simulink model "ArduCopter33StabilizeController"  (R2015b)
settings: Solver=VariableStepAuto  StartTime=0.0  StopTime=10.0  RelTol=1e-3
undefined symbols (not defined in the file): AC_ATTITUDE_RATE_RP_CONTROLLER_OUT_MAX, AC_ATTITUDE_RATE_YAW_CONTROLLER_OUT_MAX, AP_MOTORS_MAX_NUM_MOTORS, AP_MOTORS_THR_LOW_CMP_DEFAULT, AP_MOTORS_THST_MAX_DEFAULT, AP_MOTORS_YAW_HEADROOM_DEFAULT, ArduCopter, hover_throttle_pwm, init_eta, pitch_factor, RATE_PITCH_D, RATE_PITCH_FILT_HZ, RATE_PITCH_I, RATE_PITCH_IMAX, RATE_PITCH_P, RATE_ROLL_D, RATE_ROLL_FILT_HZ, RATE_ROLL_I, RATE_ROLL_IMAX, RATE_ROLL_P, RATE_YAW_D, RATE_YAW_FILT_HZ, RATE_YAW_I, RATE_YAW_IMAX, RATE_YAW_P, roll_factor, rpy_pwm_scalar, THR_MAX_DEFAULT, THR_MIN_DEFAULT, throttle_hover, throttle_pwm_scalar, THROTTLE_RADIO_LIM, yaw_factor
settings Model: Creator=jeremie  LastModifiedBy=jban039

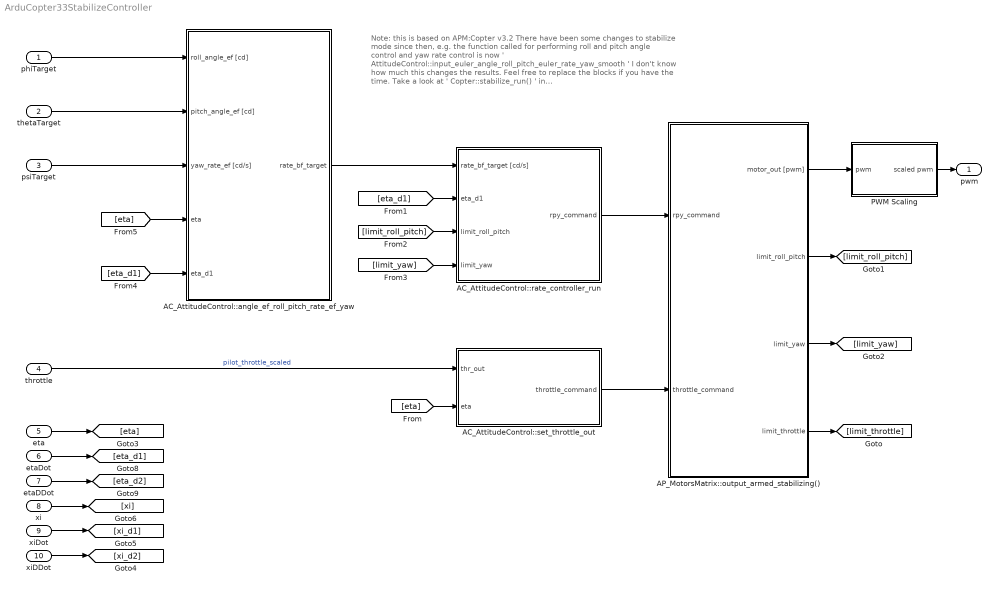
== system ArduCopter33StabilizeController ==
  note: Note: this is based on APM:Copter v3.2
      | There have been some changes to stabilize mode since then,
      | e.g. the function called for performing roll and pitch angle
      | control and yaw rate control is now
      | ' AttitudeControl::input_euler_angle_roll_pitch_euler_rate_yaw_smooth '
      | I don't know how much this changes the results. Feel free to replace the
      | blocks if you have the time.
      | Take a look at ' Copter::stabilize_run() ' in
      | ardupilot/Arducopter/control_stabilize.cpp and work from there.
  phiTarget : Inport
  thetaTarget : Inport  Port=2
  "psiTarget " : Inport  Port=3
  throttle : Inport  Port=4
  eta : Inport  Port=5
  etaDot : Inport  Port=6
  etaDDot : Inport  Port=7
  xi : Inport  Port=8
  xiDot : Inport  Port=9
  xiDDot : Inport  Port=10
  AC_AttitudeControl::angle_ef_roll_pitch_rate_ef_yaw : Subsystem
  AC_AttitudeControl::rate_controller_run : Subsystem
  AC_AttitudeControl::set_throttle_out : Subsystem
  AP_MotorsMatrix::output_armed_stabilizing() : Subsystem
  PWM Scaling : Subsystem
  pwm : Outport
  wires:
  AP_MotorsMatrix::output_armed_stabilizing()/1(motor_out [pwm]) -> PWM Scaling/1(pwm)
  xiDDot/1 -> [xi_d2]
  xiDot/1 -> [xi_d1]
  xi/1 -> [xi]
  AP_MotorsMatrix::output_armed_stabilizing()/2(limit_roll_pitch) -> [limit_roll_pitch]
  AP_MotorsMatrix::output_armed_stabilizing()/3(limit_yaw) -> [limit_yaw]
  AP_MotorsMatrix::output_armed_stabilizing()/4(limit_throttle) -> [limit_throttle]
  [eta] -> AC_AttitudeControl::set_throttle_out/2(eta)
  [eta_d1] -> AC_AttitudeControl::rate_controller_run/2(eta_d1)
  [limit_roll_pitch] -> AC_AttitudeControl::rate_controller_run/3(limit_roll_pitch)
  [limit_yaw] -> AC_AttitudeControl::rate_controller_run/4(limit_yaw)
  [eta] -> AC_AttitudeControl::angle_ef_roll_pitch_rate_ef_yaw/4(eta)
  AC_AttitudeControl::set_throttle_out/1(throttle_command) -> AP_MotorsMatrix::output_armed_stabilizing()/2(throttle_command)
  AC_AttitudeControl::rate_controller_run/1(rpy_command) -> AP_MotorsMatrix::output_armed_stabilizing()/1(rpy_command)
  etaDDot/1 -> [eta_d2]
  eta/1 -> [eta]
  etaDot/1 -> [eta_d1]
  AC_AttitudeControl::angle_ef_roll_pitch_rate_ef_yaw/1(rate_bf_target) -> AC_AttitudeControl::rate_controller_run/1(rate_bf_target [cd/s])
  [eta_d1] -> AC_AttitudeControl::angle_ef_roll_pitch_rate_ef_yaw/5(eta_d1)
  phiTarget/1 -> AC_AttitudeControl::angle_ef_roll_pitch_rate_ef_yaw/1(roll_angle_ef [cd])
  thetaTarget/1 -> AC_AttitudeControl::angle_ef_roll_pitch_rate_ef_yaw/2(pitch_angle_ef [cd])
  "psiTarget "/1 -> AC_AttitudeControl::angle_ef_roll_pitch_rate_ef_yaw/3(yaw_rate_ef [cd/s])
  throttle/1 -> AC_AttitudeControl::set_throttle_out/1(thr_out)  "pilot_throttle_scaled"
  PWM Scaling/1(scaled pwm) -> pwm/1

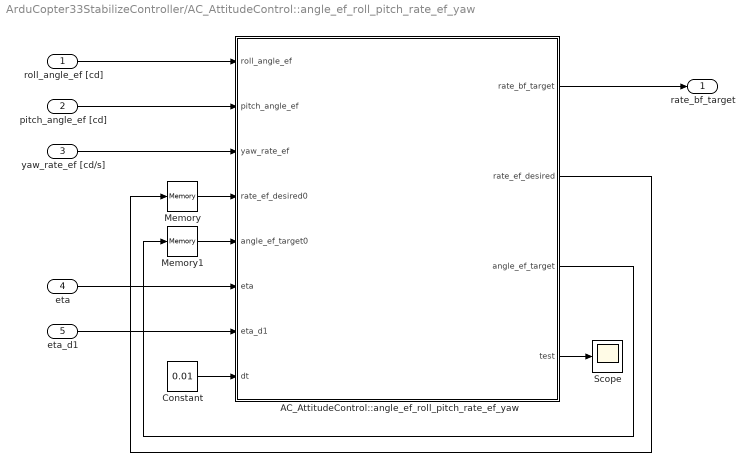
== system ArduCopter33StabilizeController/AC_AttitudeControl::angle_ef_roll_pitch_rate_ef_yaw ==
  roll_angle_ef [cd] : Inport
  pitch_angle_ef [cd] : Inport  Port=2
  yaw_rate_ef [cd/s] : Inport  Port=3
  eta : Inport  Port=4  PortDimensions=[3,1]
  eta_d1 : Inport  Port=5  PortDimensions=[3,1]
  AC_AttitudeControl::angle_ef_roll_pitch_rate_ef_yaw : MATLAB Function  TreatAsAtomicUnit=on  SystemSampleTime=0.01
  Constant : Constant  Value=0.01
  Memory : Memory  X0=[0;0;0]  InheritSampleTime=on
  Memory1 : Memory  X0=[0;0;init_eta(3)*180/pi*100]  InheritSampleTime=on
  Scope : Scope
  rate_bf_target : Outport
  wires:
  roll_angle_ef [cd]/1 -> AC_AttitudeControl::angle_ef_roll_pitch_rate_ef_yaw/1(roll_angle_ef)
  pitch_angle_ef [cd]/1 -> AC_AttitudeControl::angle_ef_roll_pitch_rate_ef_yaw/2(pitch_angle_ef)
  eta/1 -> AC_AttitudeControl::angle_ef_roll_pitch_rate_ef_yaw/6(eta)
  AC_AttitudeControl::angle_ef_roll_pitch_rate_ef_yaw/1(rate_bf_target) -> rate_bf_target/1
  AC_AttitudeControl::angle_ef_roll_pitch_rate_ef_yaw/4(test) -> Scope/1
  yaw_rate_ef [cd/s]/1 -> AC_AttitudeControl::angle_ef_roll_pitch_rate_ef_yaw/3(yaw_rate_ef)
  Memory/1 -> AC_AttitudeControl::angle_ef_roll_pitch_rate_ef_yaw/4(rate_ef_desired0)
  Memory1/1 -> AC_AttitudeControl::angle_ef_roll_pitch_rate_ef_yaw/5(angle_ef_target0)
  Constant/1 -> AC_AttitudeControl::angle_ef_roll_pitch_rate_ef_yaw/8(dt)
  AC_AttitudeControl::angle_ef_roll_pitch_rate_ef_yaw/2(rate_ef_desired) -> Memory/1
  AC_AttitudeControl::angle_ef_roll_pitch_rate_ef_yaw/3(angle_ef_target) -> Memory1/1
  eta_d1/1 -> AC_AttitudeControl::angle_ef_roll_pitch_rate_ef_yaw/7(eta_d1)

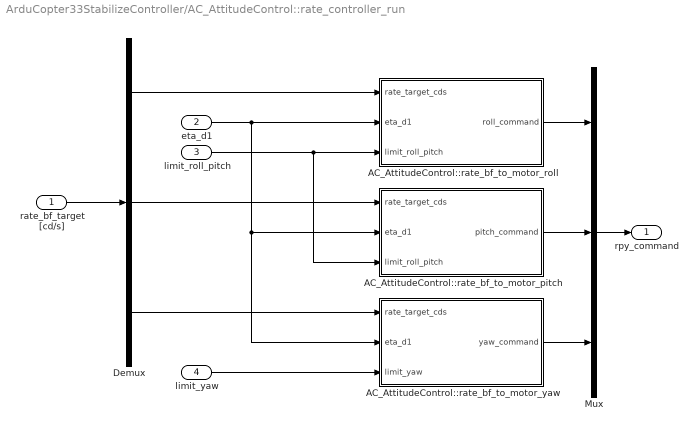
== system ArduCopter33StabilizeController/AC_AttitudeControl::rate_controller_run ==
  rate_bf_target [cd/s] : Inport
  eta_d1 : Inport  Port=2
  limit_roll_pitch : Inport  Port=3
  limit_yaw : Inport  Port=4
  AC_AttitudeControl::rate_bf_to_motor_pitch : Subsystem
  AC_AttitudeControl::rate_bf_to_motor_roll : Subsystem
  AC_AttitudeControl::rate_bf_to_motor_yaw : Subsystem
  Demux : Demux  Outputs=3
  Mux : Mux  Inputs=3
  rpy_command : Outport
  wires:
  eta_d1/1 -> AC_AttitudeControl::rate_bf_to_motor_yaw/2(eta_d1), AC_AttitudeControl::rate_bf_to_motor_pitch/2(eta_d1), AC_AttitudeControl::rate_bf_to_motor_roll/2(eta_d1)
  limit_yaw/1 -> AC_AttitudeControl::rate_bf_to_motor_yaw/3(limit_yaw)
  AC_AttitudeControl::rate_bf_to_motor_yaw/1(yaw_command) -> Mux/3
  AC_AttitudeControl::rate_bf_to_motor_pitch/1(pitch_command) -> Mux/2
  Mux/1 -> rpy_command/1
  AC_AttitudeControl::rate_bf_to_motor_roll/1(roll_command) -> Mux/1
  Demux/1 -> AC_AttitudeControl::rate_bf_to_motor_roll/1(rate_target_cds)
  Demux/2 -> AC_AttitudeControl::rate_bf_to_motor_pitch/1(rate_target_cds)
  Demux/3 -> AC_AttitudeControl::rate_bf_to_motor_yaw/1(rate_target_cds)
  rate_bf_target [cd/s]/1 -> Demux/1
  limit_roll_pitch/1 -> AC_AttitudeControl::rate_bf_to_motor_pitch/3(limit_roll_pitch), AC_AttitudeControl::rate_bf_to_motor_roll/3(limit_roll_pitch)

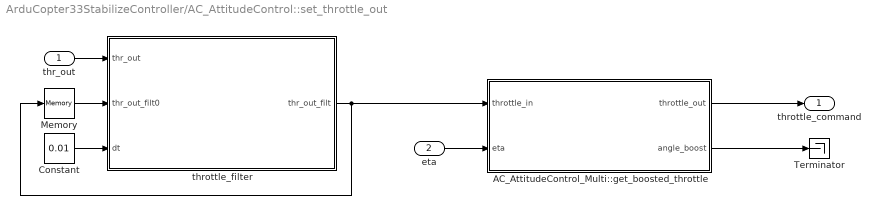
== system ArduCopter33StabilizeController/AC_AttitudeControl::set_throttle_out ==
  thr_out : Inport
  eta : Inport  Port=2
  AC_AttitudeControl_Multi::get_boosted_throttle : MATLAB Function  TreatAsAtomicUnit=on  SystemSampleTime=0.01
  Constant : Constant  Value=0.01
  Memory : Memory  X0=throttle_hover  InheritSampleTime=on
  Terminator : Terminator
  throttle_filter : MATLAB Function  TreatAsAtomicUnit=on  SystemSampleTime=0.01
  throttle_command : Outport
  wires:
  eta/1 -> AC_AttitudeControl_Multi::get_boosted_throttle/2(eta)
  AC_AttitudeControl_Multi::get_boosted_throttle/2(angle_boost) -> Terminator/1
  throttle_filter/1(thr_out_filt) -> Memory/1, AC_AttitudeControl_Multi::get_boosted_throttle/1(throttle_in)
  thr_out/1 -> throttle_filter/1(thr_out)
  Memory/1 -> throttle_filter/2(thr_out_filt0)
  Constant/1 -> throttle_filter/3(dt)
  AC_AttitudeControl_Multi::get_boosted_throttle/1(throttle_out) -> throttle_command/1

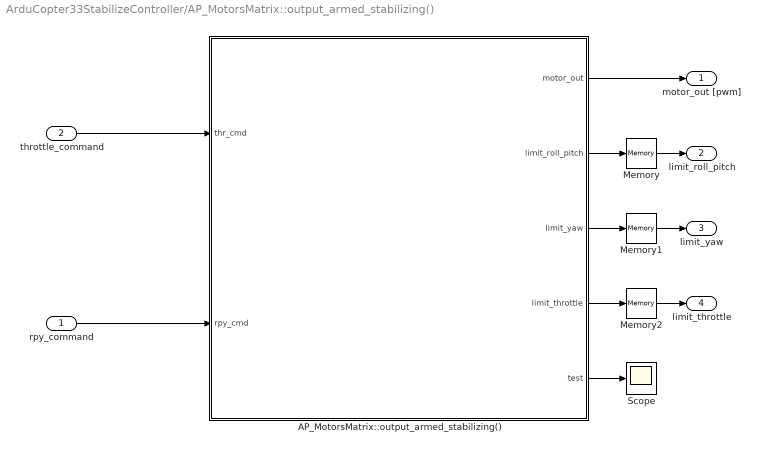
== system ArduCopter33StabilizeController/AP_MotorsMatrix::output_armed_stabilizing() ==
  rpy_command : Inport  PortDimensions=[3,1]
  throttle_command : Inport  Port=2
  AP_MotorsMatrix::output_armed_stabilizing() : MATLAB Function  TreatAsAtomicUnit=on  SystemSampleTime=0.01
  Memory : Memory  X0=false  InheritSampleTime=on
  Memory1 : Memory  X0=false  InheritSampleTime=on
  Memory2 : Memory  X0=boolean([0;0])  InheritSampleTime=on
  Scope : Scope
  motor_out [pwm] : Outport
  limit_roll_pitch : Outport  Port=2
  limit_yaw : Outport  Port=3
  limit_throttle : Outport  Port=4
  wires:
  AP_MotorsMatrix::output_armed_stabilizing()/1(motor_out) -> motor_out [pwm]/1
  rpy_command/1 -> AP_MotorsMatrix::output_armed_stabilizing()/2(rpy_cmd)
  AP_MotorsMatrix::output_armed_stabilizing()/5(test) -> Scope/1
  AP_MotorsMatrix::output_armed_stabilizing()/2(limit_roll_pitch) -> Memory/1
  AP_MotorsMatrix::output_armed_stabilizing()/3(limit_yaw) -> Memory1/1
  AP_MotorsMatrix::output_armed_stabilizing()/4(limit_throttle) -> Memory2/1
  throttle_command/1 -> AP_MotorsMatrix::output_armed_stabilizing()/1(thr_cmd)
  Memory/1 -> limit_roll_pitch/1
  Memory2/1 -> limit_throttle/1
  Memory1/1 -> limit_yaw/1

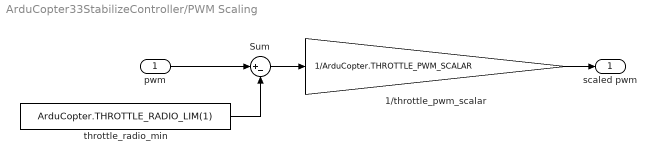
== system ArduCopter33StabilizeController/PWM Scaling ==
  pwm : Inport
  1/throttle_pwm_scalar : Gain  Gain=1/ArduCopter.THROTTLE_PWM_SCALAR
  Sum : Sum  Inputs=|+-
  throttle_radio_min : Constant  Value=ArduCopter.THROTTLE_RADIO_LIM(1)
  scaled pwm : Outport
  wires:
  1/throttle_pwm_scalar/1 -> scaled pwm/1
  throttle_radio_min/1 -> Sum/2
  Sum/1 -> 1/throttle_pwm_scalar/1
  pwm/1 -> Sum/1

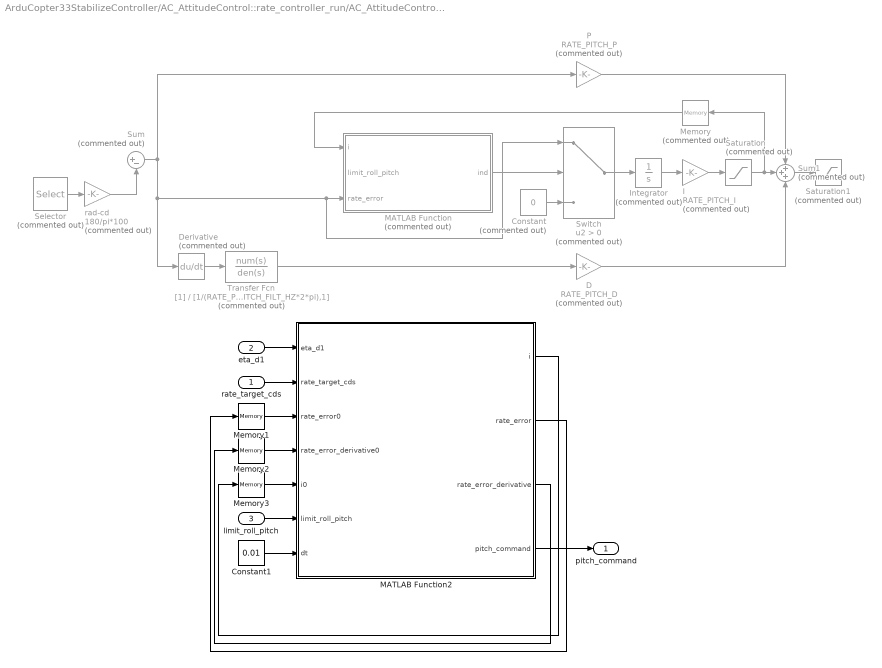
== system ArduCopter33StabilizeController/AC_AttitudeControl::rate_controller_run/AC_AttitudeControl::rate_bf_to_motor_pitch ==
  rate_target_cds : Inport
  eta_d1 : Inport  Port=2
  limit_roll_pitch : Inport  Port=3  OutDataTypeStr=boolean  PortDimensions=[1,1]
  Constant : Constant  Commented=on  Value=0
  Constant1 : Constant  Value=0.01
  D : Gain  Commented=on  Gain=RATE_PITCH_D
  Derivative : Derivative  Commented=on
  I : Gain  Commented=on  Gain=RATE_PITCH_I
  Integrator : Integrator  Commented=on
  MATLAB Function : MATLAB Function  Commented=on  TreatAsAtomicUnit=on
  MATLAB Function2 : MATLAB Function  TreatAsAtomicUnit=on  SystemSampleTime=0.01
  Memory : Memory  Commented=on  InheritSampleTime=on
  Memory1 : Memory  InheritSampleTime=on
  Memory2 : Memory  InheritSampleTime=on
  Memory3 : Memory  InheritSampleTime=on
  P : Gain  Commented=on  Gain=RATE_PITCH_P
  Saturation : Saturate  Commented=on  UpperLimit=RATE_PITCH_IMAX  LowerLimit=-RATE_PITCH_IMAX
  Saturation1 : Saturate  Commented=on  UpperLimit=AC_ATTITUDE_RATE_RP_CONTROLLER_OUT_MAX  LowerLimit=-AC_ATTITUDE_RATE_RP_CONTROLLER_OUT_MAX
  Selector : Selector  Commented=on  InputPortWidth=3  IndexOptions=Index vector (dialog)  Indices=2  OutputSizes=1
  Sum : Sum  Commented=on  Inputs=|+-
  Sum1 : Sum  Commented=on  Inputs=+++
  Switch : Switch  Commented=on  Criteria=u2 > Threshold
  Transfer Fcn : TransferFcn  Commented=on  Denominator=[1/(RATE_PITCH_FILT_HZ*2*pi),1]
  rad-cd : Gain  Commented=on  Gain=180/pi*100
  pitch_command : Outport
  wires:
  Memory1/1 -> MATLAB Function2/3(rate_error0)
  Memory3/1 -> MATLAB Function2/5(i0)
  MATLAB Function2/1(i) -> Memory3/1
  MATLAB Function2/2(rate_error) -> Memory1/1
  Constant1/1 -> MATLAB Function2/7(dt)
  Memory2/1 -> MATLAB Function2/4(rate_error_derivative0)
  MATLAB Function2/3(rate_error_derivative) -> Memory2/1
  rad-cd/1 -> Sum/2
  Integrator/1 -> I/1
  Derivative/1 -> Transfer Fcn/1
  I/1 -> Saturation/1
  Memory/1 -> MATLAB Function/1(i)
  Transfer Fcn/1 -> D/1
  Sum1/1 -> Saturation1/1
  P/1 -> Sum1/1
  D/1 -> Sum1/3
  Selector/1 -> rad-cd/1
  MATLAB Function/1(ind) -> Switch/2
  Sum/1 -> Derivative/1, Switch/1, MATLAB Function/3(rate_error), P/1
  Constant/1 -> Switch/3
  Saturation/1 -> Sum1/2, Memory/1
  Switch/1 -> Integrator/1
  MATLAB Function2/4(pitch_command) -> pitch_command/1
  limit_roll_pitch/1 -> MATLAB Function2/6(limit_roll_pitch)
  eta_d1/1 -> MATLAB Function2/1(eta_d1)
  rate_target_cds/1 -> MATLAB Function2/2(rate_target_cds)

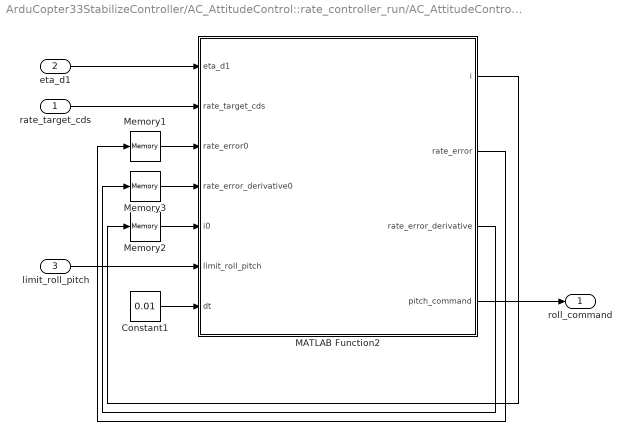
== system ArduCopter33StabilizeController/AC_AttitudeControl::rate_controller_run/AC_AttitudeControl::rate_bf_to_motor_roll ==
  rate_target_cds : Inport
  eta_d1 : Inport  Port=2
  limit_roll_pitch : Inport  Port=3  OutDataTypeStr=boolean  PortDimensions=[1,1]
  Constant1 : Constant  Value=0.01
  MATLAB Function2 : MATLAB Function  TreatAsAtomicUnit=on  SystemSampleTime=0.01
  Memory1 : Memory  InheritSampleTime=on
  Memory2 : Memory  InheritSampleTime=on
  Memory3 : Memory  InheritSampleTime=on
  roll_command : Outport
  wires:
  Memory1/1 -> MATLAB Function2/3(rate_error0)
  Memory2/1 -> MATLAB Function2/5(i0)
  MATLAB Function2/1(i) -> Memory2/1
  MATLAB Function2/2(rate_error) -> Memory1/1
  Constant1/1 -> MATLAB Function2/7(dt)
  Memory3/1 -> MATLAB Function2/4(rate_error_derivative0)
  MATLAB Function2/3(rate_error_derivative) -> Memory3/1
  MATLAB Function2/4(pitch_command) -> roll_command/1
  limit_roll_pitch/1 -> MATLAB Function2/6(limit_roll_pitch)
  eta_d1/1 -> MATLAB Function2/1(eta_d1)
  rate_target_cds/1 -> MATLAB Function2/2(rate_target_cds)

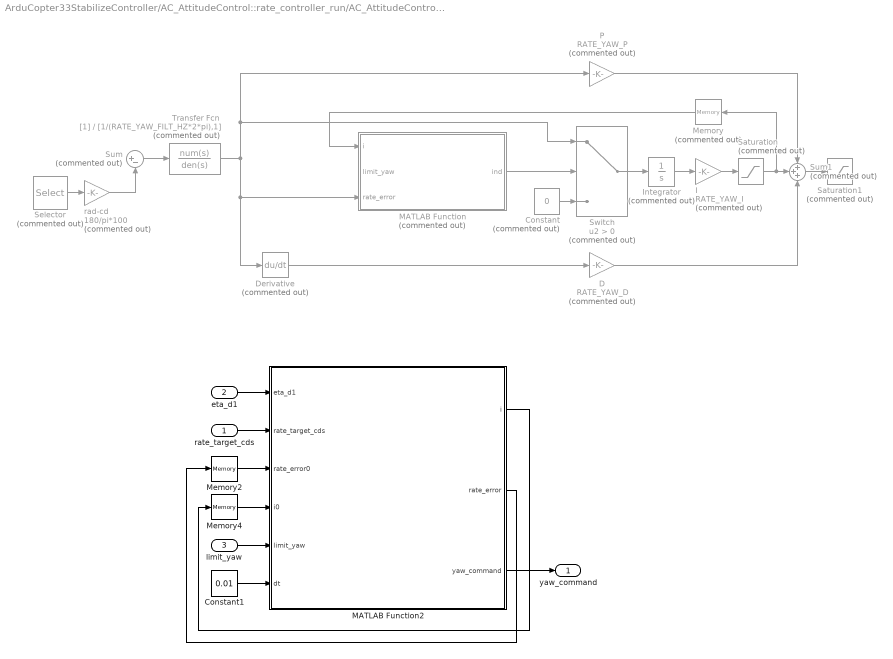
== system ArduCopter33StabilizeController/AC_AttitudeControl::rate_controller_run/AC_AttitudeControl::rate_bf_to_motor_yaw ==
  rate_target_cds : Inport
  eta_d1 : Inport  Port=2  PortDimensions=[3,1]
  limit_yaw : Inport  Port=3  OutDataTypeStr=boolean  PortDimensions=[1,1]
  Constant : Constant  Commented=on  Value=0
  Constant1 : Constant  Value=0.01
  D : Gain  Commented=on  Gain=RATE_YAW_D
  Derivative : Derivative  Commented=on
  I : Gain  Commented=on  Gain=RATE_YAW_I
  Integrator : Integrator  Commented=on
  MATLAB Function : MATLAB Function  Commented=on  TreatAsAtomicUnit=on
  MATLAB Function2 : MATLAB Function  TreatAsAtomicUnit=on  SystemSampleTime=0.01
  Memory : Memory  Commented=on  InheritSampleTime=on
  Memory2 : Memory  InheritSampleTime=on
  Memory4 : Memory  InheritSampleTime=on
  P : Gain  Commented=on  Gain=RATE_YAW_P
  Saturation : Saturate  Commented=on  UpperLimit=RATE_YAW_IMAX  LowerLimit=-RATE_YAW_IMAX
  Saturation1 : Saturate  Commented=on  UpperLimit=AC_ATTITUDE_RATE_YAW_CONTROLLER_OUT_MAX  LowerLimit=-AC_ATTITUDE_RATE_YAW_CONTROLLER_OUT_MAX
  Selector : Selector  Commented=on  InputPortWidth=3  IndexOptions=Index vector (dialog)  Indices=3  OutputSizes=1
  Sum : Sum  Commented=on  Inputs=|+-
  Sum1 : Sum  Commented=on  Inputs=+++
  Switch : Switch  Commented=on  Criteria=u2 > Threshold
  Transfer Fcn : TransferFcn  Commented=on  Denominator=[1/(RATE_YAW_FILT_HZ*2*pi),1]
  rad-cd : Gain  Commented=on  Gain=180/pi*100
  yaw_command : Outport
  wires:
  Memory2/1 -> MATLAB Function2/3(rate_error0)
  Memory4/1 -> MATLAB Function2/4(i0)
  Constant1/1 -> MATLAB Function2/6(dt)
  MATLAB Function2/1(i) -> Memory4/1
  MATLAB Function2/2(rate_error) -> Memory2/1
  rad-cd/1 -> Sum/2
  Integrator/1 -> I/1
  I/1 -> Saturation/1
  Memory/1 -> MATLAB Function/1(i)
  Derivative/1 -> D/1
  Sum1/1 -> Saturation1/1
  P/1 -> Sum1/1
  D/1 -> Sum1/3
  Selector/1 -> rad-cd/1
  MATLAB Function/1(ind) -> Switch/2
  Constant/1 -> Switch/3
  Saturation/1 -> Sum1/2, Memory/1
  Switch/1 -> Integrator/1
  Sum/1 -> Transfer Fcn/1
  Transfer Fcn/1 -> Derivative/1, MATLAB Function/3(rate_error), P/1, Switch/1
  limit_yaw/1 -> MATLAB Function2/5(limit_yaw)
  MATLAB Function2/3(yaw_command) -> yaw_command/1
  rate_target_cds/1 -> MATLAB Function2/2(rate_target_cds)
  eta_d1/1 -> MATLAB Function2/1(eta_d1)

== matlab function ArduCopter33StabilizeController/AC_AttitudeControl::set_throttle_out/AC_AttitudeControl_Multi::get_boosted_throttle ==
  data: throttle_in input; eta input; throttle_out output; THR_MIN_DEFAULT parameter; angle_boost output; throttle_pwm_scalar parameter
function [throttle_out,angle_boost] = get_boosted_throttle(throttle_in,eta,THR_MIN_DEFAULT,throttle_pwm_scalar)
%#codegen
min_throttle = THR_MIN_DEFAULT/throttle_pwm_scalar; % Is this correct?
cos_tilt = cos(eta(2))*cos(eta(1));
inverted_factor = constrain(2*cos_tilt,0,1);
boost_factor = 1/constrain(cos_tilt,0.5,1);

throttle_out = (throttle_in-min_throttle)*inverted_factor*boost_factor+min_throttle;
angle_boost = constrain(throttle_out-throttle_in,-32000,32000);

end

function constrain_val = constrain(val,min_val,max_val)
constrain_val = min([max([val,min_val]),max_val]);
end

== matlab function ArduCopter33StabilizeController/AC_AttitudeControl::angle_ef_roll_pitch_rate_ef_yaw/AC_AttitudeControl::angle_ef_roll_pitch_rate_ef_yaw ==
  data: roll_angle_ef input; pitch_angle_ef input; yaw_rate_ef input; rate_ef_desired0 input; angle_ef_target0 input; eta input; eta_d1 input; dt input; STABILIZE_ROLL_P parameter; STABILIZE_PITCH_P parameter; STABILIZE_YAW_P parameter; AC_ATTITUDE_CONTROL_ACCEL_RP_MAX_DEFAULT parameter; AC_ATTITUDE_ANGLE_CONTROLLER_ANGLE_MAX parameter; AC_ATTITUDE_CONTROL_ACCEL_Y_MAX_DEFAULT parameter; AC_ATTITUDE_ACCEL_RP_CONTROLLER_MIN parameter; AC_ATTITUDE_ACCEL_RP_CONTROLLER_MAX parameter; AC_ATTITUDE_ACCEL_Y_CONTROLLER_MIN parameter; AC_ATTITUDE_ACCEL_Y_CONTROLLER_MAX parameter; rate_bf_target output; rate_ef_desired output; angle_ef_target output; test output; AC_ATTITUDE_RATE_STAB_YAW_OVERSHOOT_ANGLE_MAX parameter
function [rate_bf_target,rate_ef_desired,angle_ef_target,test] = angle_ef_roll_pitch_rate_ef_yaw(roll_angle_ef,pitch_angle_ef,yaw_rate_ef,...
    rate_ef_desired0,angle_ef_target0,...
    eta,eta_d1,dt,...
    STABILIZE_ROLL_P,STABILIZE_PITCH_P,STABILIZE_YAW_P,...
    AC_ATTITUDE_CONTROL_ACCEL_RP_MAX_DEFAULT,...
    AC_ATTITUDE_ANGLE_CONTROLLER_ANGLE_MAX,AC_ATTITUDE_CONTROL_ACCEL_Y_MAX_DEFAULT,...
    AC_ATTITUDE_ACCEL_RP_CONTROLLER_MIN,AC_ATTITUDE_ACCEL_RP_CONTROLLER_MAX,...
    AC_ATTITUDE_ACCEL_Y_CONTROLLER_MIN,AC_ATTITUDE_ACCEL_Y_CONTROLLER_MAX,...
    AC_ATTITUDE_RATE_STAB_YAW_OVERSHOOT_ANGLE_MAX)
%#codegen
angle_kP = [STABILIZE_ROLL_P;
    STABILIZE_PITCH_P;
    STABILIZE_YAW_P];
accel_max = [AC_ATTITUDE_CONTROL_ACCEL_RP_MAX_DEFAULT;
    AC_ATTITUDE_CONTROL_ACCEL_RP_MAX_DEFAULT;
    AC_ATTITUDE_CONTROL_ACCEL_Y_MAX_DEFAULT];

% convert to centi-degrees
eta_cd = eta*(180/pi*100);

% initialise vectors
angle_ef_target = zeros(3,1); % [roll;pitch;yaw]
angle_ef_error = zeros(3,1);  % [roll;pitch;yaw]
rate_ef_desired = zeros(3,1);

% set earth-frame angle targets for roll and pitch and calculate angle error
angle_ef_target(1) = constrain(roll_angle_ef,-AC_ATTITUDE_ANGLE_CONTROLLER_ANGLE_MAX,AC_ATTITUDE_ANGLE_CONTROLLER_ANGLE_MAX);
angle_ef_error(1) = wrap_180_cd(angle_ef_target(1)-eta_cd(1));

angle_ef_target(2) = constrain(pitch_angle_ef,-AC_ATTITUDE_ANGLE_CONTROLLER_ANGLE_MAX,AC_ATTITUDE_ANGLE_CONTROLLER_ANGLE_MAX);
angle_ef_error(2) = wrap_180_cd(angle_ef_target(2)-eta_cd(2));

if (AC_ATTITUDE_CONTROL_ACCEL_Y_MAX_DEFAULT > 0)
    % set earth-frame feed forward rate for yaw
    rate_change_limit = AC_ATTITUDE_CONTROL_ACCEL_Y_MAX_DEFAULT*dt;
    rate_change = yaw_rate_ef-rate_ef_desired0(3);
    rate_change = constrain(rate_change,-rate_change_limit,rate_change_limit);
    rate_ef_desired(3) = rate_ef_desired0(3)+rate_change;
    % calculate yaw target angle and angle error
    [angle_ef_error(3),angle_ef_target(3)] = ...
        update_ef_yaw_angle_and_error(angle_ef_target0(3),...
        yaw_rate_ef,eta_cd(3),AC_ATTITUDE_RATE_STAB_YAW_OVERSHOOT_ANGLE_MAX,dt);
else
    % set yaw feed forward to zero
    rate_ef_desired(3) = yaw_rate_ef;
    % calculate yaw target angle and angle error
    [angle_ef_error(3),angle_ef_target(3)] = ...
        update_ef_yaw_angle_and_error(angle_ef_target0(3),...
        yaw_rate_ef,eta_cd(3),AC_ATTITUDE_RATE_STAB_YAW_OVERSHOOT_ANGLE_MAX,dt);
end
test = angle_ef_target0(3)-eta_cd(3);

% convert earth-frame angle errors to body-frame angle errors
angle_bf_error = frame_conversion_ef_to_bf(angle_ef_error,eta);

% convert body-frame angle errors to body-frame rate targets
rate_bf_target = update_rate_bf_targets(angle_bf_error,eta_d1,...
    angle_kP,accel_max,...
    AC_ATTITUDE_ACCEL_RP_CONTROLLER_MIN,AC_ATTITUDE_ACCEL_RP_CONTROLLER_MAX,...
    AC_ATTITUDE_ACCEL_Y_CONTROLLER_MIN,AC_ATTITUDE_ACCEL_Y_CONTROLLER_MAX); % CHECK YAW!!!

% set roll and pitch feed forward to zero
rate_ef_desired(1) = 0;
rate_ef_desired(2) = 0;

% convert earth-frame feed forward rates to body-frame feed forward rates
rate_bf_desired = frame_conversion_ef_to_bf(rate_ef_desired,eta);
rate_bf_target = rate_bf_target+rate_bf_desired;

end

%%
function constrain_val = constrain(val,min_val,max_val)
constrain_val = min([max([val,min_val]),max_val]);
end

function wrap_val = wrap_180_cd(val)
if (val > 360000 || val < -36000)
    % for very large numbers use modulus
    wrap_val = mod(val,36000);
else
    wrap_val = val;
end
while (wrap_val > 18000)
    wrap_val = wrap_val-36000;
end
while (wrap_val < -18000)
    wrap_val = wrap_val+36000;
end
end

function wrap_val = wrap_360_cd(val)
if (val >= 720000 || val < -360000)
    % for very large numbers use modulus
    wrap_val = mod(val,36000);
else
    wrap_val = val;
end
while (wrap_val >= 36000)
    wrap_val = wrap_val-36000;
end
while (wrap_val < 0)
    wrap_val = wrap_val+36000;
end
end

function [angle_ef_error_z,angle_ef_target_z] = update_ef_yaw_angle_and_error(angle_ef_target_z,yaw_rate_ef,yaw_sensor,overshoot_max,dt)
% calculate angle error with maximum of +- max angle overshoot
angle_ef_error_z = wrap_180_cd(angle_ef_target_z-yaw_sensor);
angle_ef_error_z = constrain(angle_ef_error_z,-overshoot_max,overshoot_max);

% update yaw angle target to be within max angle overshoot of our current heading
angle_ef_target_z = angle_ef_error_z+yaw_sensor;

% increment the yaw angle target
angle_ef_target_z = angle_ef_target_z+yaw_rate_ef*dt;
angle_ef_target_z = wrap_360_cd(angle_ef_target_z);
end

function bf_vector = frame_conversion_ef_to_bf(ef_vector,eta)
bf_vector = [1,0,-sin(eta(2));
    0,cos(eta(1)),sin(eta(1))*cos(eta(2));
    0,-sin(eta(1)),cos(eta(1))*cos(eta(2))]*ef_vector;
end

function rate_bf_target = update_rate_bf_targets(angle_bf_error,eta_d1,...
    angle_kP,accel_max,...
    AC_ATTITUDE_ACCEL_RP_CONTROLLER_MIN,AC_ATTITUDE_ACCEL_RP_CONTROLLER_MAX,...
    AC_ATTITUDE_ACCEL_Y_CONTROLLER_MIN,AC_ATTITUDE_ACCEL_Y_CONTROLLER_MAX)
rate_bf_target = zeros(3,1);

% stab roll calculation
% constrain roll rate request
rate_bf_target(1) = sqrt_controller(angle_bf_error(1),angle_kP(1),...
    constrain(accel_max(1)/2,AC_ATTITUDE_ACCEL_RP_CONTROLLER_MIN,AC_ATTITUDE_ACCEL_RP_CONTROLLER_MAX));

% stab pitch calculation
% constrain pitch rate request
rate_bf_target(2) = sqrt_controller(angle_bf_error(2),angle_kP(2),...
    constrain(accel_max(2)/2,AC_ATTITUDE_ACCEL_RP_CONTROLLER_MIN,AC_ATTITUDE_ACCEL_RP_CONTROLLER_MAX));

% stab yaw calculation
% constrain yaw rate request
rate_bf_target(3) = sqrt_controller(angle_bf_error(3),angle_kP(3),...
    constrain(accel_max(3)/2,AC_ATTITUDE_ACCEL_Y_CONTROLLER_MIN,AC_ATTITUDE_ACCEL_Y_CONTROLLER_MAX));

% include roll and pitch rate required to account for precession of the desired attitude about the body frame yaw axes
rate_bf_target(1) = rate_bf_target(1)+angle_bf_error(2)*eta_d1(3);
rate_bf_target(2) = rate_bf_target(2)-angle_bf_error(1)*eta_d1(3);
end

% AC_AttitudeControl::sqrt_controller
function u = sqrt_controller(error,p,second_ord_lim)
if (second_ord_lim == 0 || p == 0)
    u = error*p;
    return
end

linear_dist = second_ord_lim/p^2;

if (error > linear_dist)
    u = safe_sqrt(2*second_ord_lim*(error-(linear_dist/2)));
    return
elseif (error < -linear_dist)
    u = -safe_sqrt(2*second_ord_lim*(-error-(linear_dist/2)));
    return
else
    u = error*p;
    return
end
end

function v = safe_sqrt(u)
if (u < 0)
    v = 0;
else
    v = sqrt(u);
end
end

== matlab function ArduCopter33StabilizeController/AC_AttitudeControl::rate_controller_run/AC_AttitudeControl::rate_bf_to_motor_pitch/MATLAB Function2 ==
  data: eta_d1 input; i output; rate_target_cds input; rate_error0 input; rate_error_derivative0 input; i0 input; limit_roll_pitch input; rate_error output; rate_error_derivative output; pitch_command output; dt input; RATE_PITCH_P parameter; RATE_PITCH_I parameter; RATE_PITCH_D parameter; AC_ATTITUDE_RATE_RP_CONTROLLER_OUT_MAX parameter; RATE_PITCH_IMAX parameter; RATE_PITCH_FILT_HZ parameter
function [i,rate_error,rate_error_derivative,pitch_command] = ...
    rate_bf_to_motor_pitch(eta_d1,rate_target_cds,...
    rate_error0,rate_error_derivative0,i0,limit_roll_pitch,dt,...
    RATE_PITCH_P,RATE_PITCH_I,RATE_PITCH_D,AC_ATTITUDE_RATE_RP_CONTROLLER_OUT_MAX,...
    RATE_PITCH_IMAX,RATE_PITCH_FILT_HZ)
%#codegen

% get current rate
current_rate = eta_d1(2)*(180/pi*100); % BODY OR EARTH FRAME?

% calculate error and call pid controller
rate_error = rate_target_cds-current_rate;

% calculate and filter derivative
rate_error_derivative = set_input_filter_d(rate_error,rate_error0,rate_error_derivative0,RATE_PITCH_FILT_HZ,dt);

% get p value
p = RATE_PITCH_P*rate_error;

% get i term
i = i0;

% update i term as long as we haven't breached the limits or the i term
% will certainly reduce
if (~limit_roll_pitch || ((i > 0 && rate_error < 0) || (i < 0 && rate_error > 0)))
    i = get_i(RATE_PITCH_I,i,rate_error,RATE_PITCH_IMAX,dt);
end

% get d value
d = RATE_PITCH_D*rate_error_derivative;

% constrain output and return
pitch_command = constrain(p+i+d,-AC_ATTITUDE_RATE_RP_CONTROLLER_OUT_MAX,AC_ATTITUDE_RATE_RP_CONTROLLER_OUT_MAX);

end

%%
function con_val = constrain(val,min_val,max_val)
con_val = min([max([val,min_val]),max_val]);
end

function i = get_i(ki,i0,error,imax,dt)
i = i0+ki*error*dt;
if (i < -imax)
    i = -imax;
elseif (i > imax)
    i = imax;
end
end

function derivative = set_input_filter_d(input,input0,derivative0,filt_cutoff,dt)
rc = 1/(2*pi*filt_cutoff);
alpha = dt/(dt+rc);
derivative = (input-input0)/dt;
derivative = derivative0+alpha*(derivative-derivative0);
end

== matlab function ArduCopter33StabilizeController/AC_AttitudeControl::rate_controller_run/AC_AttitudeControl::rate_bf_to_motor_yaw/MATLAB Function2 ==
  data: eta_d1 input; i output; rate_target_cds input; rate_error0 input; i0 input; limit_yaw input; dt input; RATE_YAW_P parameter; RATE_YAW_I parameter; RATE_YAW_D parameter; rate_error output; yaw_command output; AC_ATTITUDE_RATE_YAW_CONTROLLER_OUT_MAX parameter; RATE_YAW_IMAX parameter; RATE_YAW_FILT_HZ parameter
function [i,rate_error,yaw_command] = ...
    rate_bf_to_motor_yaw(eta_d1,rate_target_cds,rate_error0,i0,limit_yaw,dt,...
    RATE_YAW_P,RATE_YAW_I,RATE_YAW_D,AC_ATTITUDE_RATE_YAW_CONTROLLER_OUT_MAX,...
    RATE_YAW_IMAX,RATE_YAW_FILT_HZ)
%#codegen

% get current rate
current_rate = eta_d1(3)*(180/pi*100); % BODY OR EARTH FRAME?

% calculate error and call pid controller
rate_error = rate_target_cds-current_rate;

% filter rate_error and calculate derivative
[rate_error,derivative_error] = set_input_filter_all(rate_error,rate_error0,RATE_YAW_FILT_HZ,dt);

% get p value
p = RATE_YAW_P*rate_error;

% get i term
i = i0;

% update i term as long as we haven't breached the limits or the i term
% will certainly reduce
if (~limit_yaw || ((i > 0 && rate_error < 0) || (i < 0 && rate_error > 0)))
    i = get_i(RATE_YAW_I,i,rate_error,RATE_YAW_IMAX,dt);
end

% get d value
d = RATE_YAW_D*derivative_error;

% constrain output and return
yaw_command = constrain(p+i+d,-AC_ATTITUDE_RATE_YAW_CONTROLLER_OUT_MAX,AC_ATTITUDE_RATE_YAW_CONTROLLER_OUT_MAX);

end

%%
function con_val = constrain(val,min_val,max_val)
con_val = min([max([val,min_val]),max_val]);
end

function i = get_i(ki,i0,error,imax,dt)
i = i0+ki*error*dt;
if (i < -imax)
    i = -imax;
elseif (i > imax)
    i = imax;
end
end

function [output,derivative] = set_input_filter_all(input,input0,filt_cutoff,dt)
rc = 1/(2*pi*filt_cutoff);
alpha = dt/(dt+rc);
input_filt_change = alpha*(input-input0);
output = input0+input_filt_change;
derivative = input_filt_change/dt;
end

== matlab function ArduCopter33StabilizeController/AC_AttitudeControl::rate_controller_run/AC_AttitudeControl::rate_bf_to_motor_pitch/MATLAB Function ==
  data: i input; ind output; limit_roll_pitch input; rate_error input
function ind = check_limits(i,limit_roll_pitch,rate_error)
%#codegen
ind = 0;
if (~limit_roll_pitch || ((i > 0 && rate_error < 0) || (i < 0 && rate_error > 0)))
   ind = 1; 
end
end

== matlab function ArduCopter33StabilizeController/AC_AttitudeControl::rate_controller_run/AC_AttitudeControl::rate_bf_to_motor_yaw/MATLAB Function ==
  data: i input; ind output; limit_yaw input; rate_error input
function ind = check_limits(i,limit_yaw,rate_error)
%#codegen
ind = 0;
if (~limit_yaw || ((i > 0 && rate_error < 0) || (i < 0 && rate_error > 0)))
   ind = 1; 
end
end

== matlab function ArduCopter33StabilizeController/AC_AttitudeControl::set_throttle_out/throttle_filter ==
  data: thr_out input; thr_out_filt0 input; dt input; POSCONTROL_THROTTLE_CUTOFF_FREQ parameter; thr_out_filt output
function thr_out_filt = fcn(thr_out,thr_out_filt0,dt,POSCONTROL_THROTTLE_CUTOFF_FREQ)
%#codegen
% Calculate alpha
rc = 1/(2*pi*POSCONTROL_THROTTLE_CUTOFF_FREQ);
alpha = dt/(dt+rc);
thr_out_filt = thr_out_filt0+alpha*double(thr_out-thr_out_filt0);
end

== matlab function ArduCopter33StabilizeController/AC_AttitudeControl::rate_controller_run/AC_AttitudeControl::rate_bf_to_motor_roll/MATLAB Function2 ==
  data: eta_d1 input; i output; rate_target_cds input; rate_error0 input; rate_error_derivative0 input; i0 input; limit_roll_pitch input boolean size=[1,1]; rate_error output; rate_error_derivative output; pitch_command output; dt input; RATE_ROLL_P parameter; RATE_ROLL_I parameter; RATE_ROLL_D parameter; AC_ATTITUDE_RATE_RP_CONTROLLER_OUT_MAX parameter; RATE_ROLL_IMAX parameter; RATE_ROLL_FILT_HZ parameter
function [i,rate_error,rate_error_derivative,pitch_command] = ...
    rate_bf_to_motor_roll(eta_d1,rate_target_cds,...
    rate_error0,rate_error_derivative0,i0,limit_roll_pitch,dt,...
    RATE_ROLL_P,RATE_ROLL_I,RATE_ROLL_D,AC_ATTITUDE_RATE_RP_CONTROLLER_OUT_MAX,...
    RATE_ROLL_IMAX,RATE_ROLL_FILT_HZ)
%#codegen

% get current rate
current_rate = eta_d1(1)*(180/pi*100); % BODY OR EARTH FRAME?

% calculate error and call pid controller
rate_error = rate_target_cds-current_rate;

% calculate and filter derivative
rate_error_derivative = set_input_filter_d(rate_error,rate_error0,rate_error_derivative0,RATE_ROLL_FILT_HZ,dt);

% get p value
p = RATE_ROLL_P*rate_error;

% get i term
i = i0;

% update i term as long as we haven't breached the limits or the i term
% will certainly reduce
if (~limit_roll_pitch || ((i > 0 && rate_error < 0) || (i < 0 && rate_error > 0)))
    i = get_i(RATE_ROLL_I,i,rate_error,RATE_ROLL_IMAX,dt);
end

% get d value
d = RATE_ROLL_D*rate_error_derivative;

% constrain output and return
pitch_command = constrain(p+i+d,-AC_ATTITUDE_RATE_RP_CONTROLLER_OUT_MAX,AC_ATTITUDE_RATE_RP_CONTROLLER_OUT_MAX);

end

%%
function con_val = constrain(val,min_val,max_val)
con_val = min([max([val,min_val]),max_val]);
end

function i = get_i(ki,i0,error,imax,dt)
i = i0+ki*error*dt;
if (i < -imax)
    i = -imax;
elseif (i > imax)
    i = imax;
end
end

function derivative = set_input_filter_d(input,input0,derivative0,filt_cutoff,dt)
rc = 1/(2*pi*filt_cutoff);
alpha = dt/(dt+rc);
derivative = (input-input0)/dt;
derivative = derivative0+alpha*(derivative-derivative0);
end

== matlab function ArduCopter33StabilizeController/AP_MotorsMatrix::output_armed_stabilizing()/AP_MotorsMatrix::output_armed_stabilizing() ==
  data: thr_cmd input; rpy_cmd input; THROTTLE_RADIO_LIM parameter; THR_MIN_DEFAULT parameter; THR_MAX_DEFAULT parameter; AP_MOTORS_THR_LOW_CMP_DEFAULT parameter; AP_MOTORS_YAW_HEADROOM_DEFAULT parameter; hover_throttle_pwm parameter; motor_out output size=4; throttle_pwm_scalar parameter size=1; rpy_pwm_scalar parameter; roll_factor parameter; pitch_factor parameter; yaw_factor parameter; limit_roll_pitch output; limit_yaw output; limit_throttle output; AP_MOTORS_THST_MAX_DEFAULT parameter; AP_MOTORS_MAX_NUM_MOTORS parameter; test output
function [motor_out,limit_roll_pitch, limit_yaw,limit_throttle,test]...
    = output_armed_stabilizing(thr_cmd,rpy_cmd,...
    THROTTLE_RADIO_LIM,THR_MIN_DEFAULT,THR_MAX_DEFAULT,AP_MOTORS_THR_LOW_CMP_DEFAULT,...
    AP_MOTORS_YAW_HEADROOM_DEFAULT,...
    hover_throttle_pwm,...
    throttle_pwm_scalar,rpy_pwm_scalar,...
    roll_factor,pitch_factor,yaw_factor,...
    AP_MOTORS_THST_MAX_DEFAULT,...
    AP_MOTORS_MAX_NUM_MOTORS)
%#codegen
throttle_radio_min = THROTTLE_RADIO_LIM(1);
throttle_radio_max = THROTTLE_RADIO_LIM(2);
min_throttle = THR_MIN_DEFAULT;
max_throttle = THR_MAX_DEFAULT;
%fx_factor = fxy_factor(:,1);
%fy_factor = fxy_factor(:,2);
throttle_thr_mix = AP_MOTORS_THR_LOW_CMP_DEFAULT;
yaw_headroom = AP_MOTORS_YAW_HEADROOM_DEFAULT;
thrust_curve_max = AP_MOTORS_THST_MAX_DEFAULT;
lift_max = 1;

% -------------------------------------------------------------------------
out_min_pwm = throttle_radio_min+min_throttle;
% out_min_pwm = throttle_radio_min+min_throttle*throttle_pwm_scalar; % JC: Alternative calculation?
out_max_pwm = throttle_radio_max;
out_mid_pwm = (out_min_pwm+out_max_pwm)/2;
rpy_scale = 1;              % This is used to scale the roll, pitch and yaw to fit within the motor limits

thr_adj = 0;        % The difference between the pilot's desired throttle and out_best_thr_pwm (the throttle that is actually provided) % WHERE IS THIS CALCULATED - CHECK!!!

% Initialise limit flags
limit_roll_pitch = false;
limit_yaw = false;
limit_throttle = false(2,1); % [lower,upper]

% Ensure throttle is within bounds of 0 to 1000
thr_in_min = rel_pwm_to_thr_range(min_throttle,throttle_pwm_scalar);
% thr_in_min = min_throttle; % Limit thr_cmd to 130-1000?
if (thr_cmd <= thr_in_min)
    thr_cmd = thr_in_min;
    limit_throttle(1) = true;
end
if (thr_cmd >= max_throttle)
    thr_cmd = max_throttle;
    limit_throttle(2) = true;
end

roll_pwm = rpy_cmd(1)*rpy_pwm_scalar;
pitch_pwm = rpy_cmd(2)*rpy_pwm_scalar;
yaw_pwm = rpy_cmd(3)*rpy_pwm_scalar;
throttle_radio_output = thr_cmd*throttle_pwm_scalar+throttle_radio_min;
%fx_pwm = fxy_cmd(1)*fxy_pwm_scalar;
%fy_pwm = fxy_cmd(2)*fxy_pwm_scalar;

% Calculate roll and pitch for each motor
rpy_out = roll_pwm*roll_factor+pitch_pwm*pitch_factor;
% Add fxy command for each motor
% rpy_out = rpy_out+fx_pwm*fx_factor+fy_pwm*fy_factor;
% Record high/low command
rpy_low = min(rpy_out);
rpy_high = max(rpy_out);

% KS: bypass this adjustment of throttle - need to resolve why only out_mid_pwm is the output for high input throttle settings
% calculate throttle that gives most possible room for yaw (range 1000 ~ 2000) which is the lower of:
%      1. mid throttle - average of highest and lowest motor (this would give the maximum possible room margin above the highest motor and below the lowest)
%      2. the higher of:
%            a) the pilot's throttle input
%            b) the mid point between the pilot's input throttle and hover-throttle
%      Situation #2 ensure we never increase the throttle above hover throttle unless the pilot has commanded this.
%      Situation #2b allows us to raise the throttle above what the pilot commanded but not so far that it would actually cause the copter to rise.
%      We will choose #1 (the best throttle for yaw control) if that means reducing throttle to the motors (i.e. we favour reducing throttle *because* it provides better yaw control)
%      We will choose #2 (a mix of pilot and hover throttle) only when the throttle is quite low.  We favour reducing throttle instead of better yaw control because the pilot has commanded it
motor_mid = (rpy_low+rpy_high)/2;
out_best_thr_pwm = min([out_mid_pwm-motor_mid,...
    max([throttle_radio_output,...
    throttle_radio_output*max([0,1-throttle_thr_mix])+hover_throttle_pwm*throttle_thr_mix])]);
% out_best_thr_pwm = throttle_radio_output;   % KS

% calculate amount of yaw we can fit into the throttle range
% this is always equal to or less than the requested yaw from the pilot or rate controller
yaw_allowed = min([out_max_pwm-out_best_thr_pwm,out_best_thr_pwm-out_min_pwm])-(rpy_high-rpy_low)/2;
yaw_allowed = max([yaw_allowed,yaw_headroom]);

if (yaw_pwm >= 0)
    % If yawing right
    if (yaw_allowed > yaw_pwm)
        yaw_allowed = yaw_pwm;
    else
        limit_yaw = true;
    end
else
    % If yawing left
    yaw_allowed = -yaw_allowed;
    if (yaw_allowed < yaw_pwm)
        yaw_allowed = yaw_pwm;
    else
        limit_yaw = true;
    end
end

% add yaw to intermediate numbers for each motor
rpy_out = rpy_out+yaw_allowed*yaw_factor;
% Record lowest roll+pitch+yaw command
rpy_low = min(rpy_out);
rpy_high = max(rpy_out);

% Check everything fits
thr_adj_max = max([out_max_pwm-(out_best_thr_pwm+rpy_high),0]);

% If we are increasing thr throttle (situation #2 above)...
if (thr_adj > 0)
    % increase throttle as close as possible to requested throttle without going over out_max_pwm
    if (thr_adj > thr_adj_max)
        thr_adj = thr_adj_max;
        % we haven't even been able to apply full throttle command
        limit_throttle(2) = true;
    end
elseif (thr_adj < 0)
    % decrease throttle as close as possible to requested throttle without going under out_min_pwm or over out_max_pwm
    thr_adj_min = min([out_min_pwm-(out_best_thr_pwm+rpy_low),0]);
    if (thr_adj > thr_adj_max)
        thr_adj = thr_adj_max;
        limit_throttle(2) = true;
    end
    if (thr_adj < thr_adj_min)
        thr_adj = thr_adj_min;
        limit_throttle(1) = true; % JC: Added
    end
end

% do we need to reduce roll, pitch, yaw command
if ((rpy_low+out_best_thr_pwm)+thr_adj < out_min_pwm)
    % protect against divide by zero
    if (rpy_low ~= 0)
        rpy_scale = (out_min_pwm-thr_adj-out_best_thr_pwm)/rpy_low;
    end
    % we haven't even been able to apply full roll, pitch and minimal yaw without scaling
    limit_roll_pitch = true;
    limit_yaw = true;
elseif ((rpy_high+out_best_thr_pwm)+thr_adj > out_max_pwm)
    if (rpy_low ~= 0)
        rpy_scale = (out_max_pwm-thr_adj-out_best_thr_pwm)/rpy_high;
    end
    % we haven't even been able to apply full roll, pitch and minimal yaw without scaling
    limit_roll_pitch = true;
    limit_yaw = true;
end

% NEED TO CHANGE SCALING TO ALLOW NON-SYMMETRICAL MOTOR COMMANDS...

% add scaled roll, pitch, constrained yaw and throttle for each motor
motor_out = out_best_thr_pwm+thr_adj+rpy_scale*rpy_out;
test = [motor_out(2:3)];

% apply thrust curve and voltage_scaling (is this needed?)
% for i=1:AP_MOTORS_MAX_NUM_MOTORS
%     motor_out(i) = apply_thrust_curve_and_volt_scaling(motor_out(i),out_min_pwm,out_max_pwm,...
%         thrust_curve_param,thrust_curve_max,lift_max,batt_voltage_filt);
% end

% clip motor output if required (shouldn't be)
for i=1:AP_MOTORS_MAX_NUM_MOTORS
    motor_out(i) = constrain(motor_out(i),out_min_pwm,out_max_pwm);
end
end

%% SUBFUNCTIONS
function thr_in_min = rel_pwm_to_thr_range(min_throttle,throttle_pwm_scalar)
thr_in_min = min_throttle/throttle_pwm_scalar;
end

function compensation_gain = get_compensation_gain
compensation_gain = 1;
end

function constrained_val = constrain(val,min_val,max_val)
constrained_val = min([max([val,min_val]),max_val]);
end

function pwm_out_scaled = apply_thrust_curve_and_volt_scaling(pwm_out,pwm_min,pwm_max,...
    thrust_curve_param,thrust_curve_max,...
    lift_max,batt_voltage_filt)
thrust_curve_expo = thrust_curve_param(2);
% convert to 0.0 to 1.0 ratio
throttle_ratio = (pwm_out-pwm_min)/(pwm_max-pwm_min);

% apply thrust curve - domain 0.0 to 1.0, range 0.0 to 1.0
if (thrust_curve_expo > 0)
    throttle_ratio = ((thrust_curve_expo-1)+...
        safe_sqrt((1-thrust_curve_expo)^2+4*thrust_curve_expo*lift_max*throttle_ratio))/...
        (2*thrust_curve_expo*batt_voltage_filt);
end

% scale to maximum thrust point
throttle_ratio = throttle_ratio*thrust_curve_max;

% convert back to pwm range, constrain and return
pwm_out_scaled = throttle_ratio*(pwm_max-pwm_min)+pwm_min;
pwm_out_scaled = constrain(pwm_out_scaled,pwm_min,(pwm_max-pwm_min)*thrust_curve_max+pwm_min);

end

function ret = safe_sqrt(v)
if (v < 0)
    ret = 0;
else
    ret = sqrt(v);
end
end
